simulink model "VCOs"  (R2019b)
settings: Solver=FixedStepAuto  StartTime=0.0  StopTime=simt  FixedStep=sampt  RelTol=1e-3
model workspace (MAT data in the model file):
  VCOctrl = 1
  Vc = 2.421875
  VcoParamResultTable = [nan nan]
  frequencyVector = [nan nan nan nan nan nan nan nan nan nan]
  kvcoVector = [nan nan nan nan nan nan nan nan nan]
  myParam = Simulink.Parameter
  myParam.Value = 2
  myParam.DataType = 'auto'
  myParam.Min = 0
  myParam.Max = 5
  myParam.Dimensions = [1 1]
  myParam2 = 2
  quiescentFreq = nan
  vctrlVector = [1 1.44 1.89 2.33 2.78 3.22 3.67 4.11 4.56 5]
values from neighbouring files (symbols this model uses):
  simt = 1/100000    (= 1e-05)    [FreqSpectrum.m]    (also in VCO.m)
libraries: impairlib x1, simulink x1, msbPllFoundation x1
settings Model: OrderedModelArguments=off  Creator=lfbarrag  LastModifiedBy=Luis Barragan
settings DataIOCC: SaveFormat=Array  ReturnWorkspaceOutputs=off

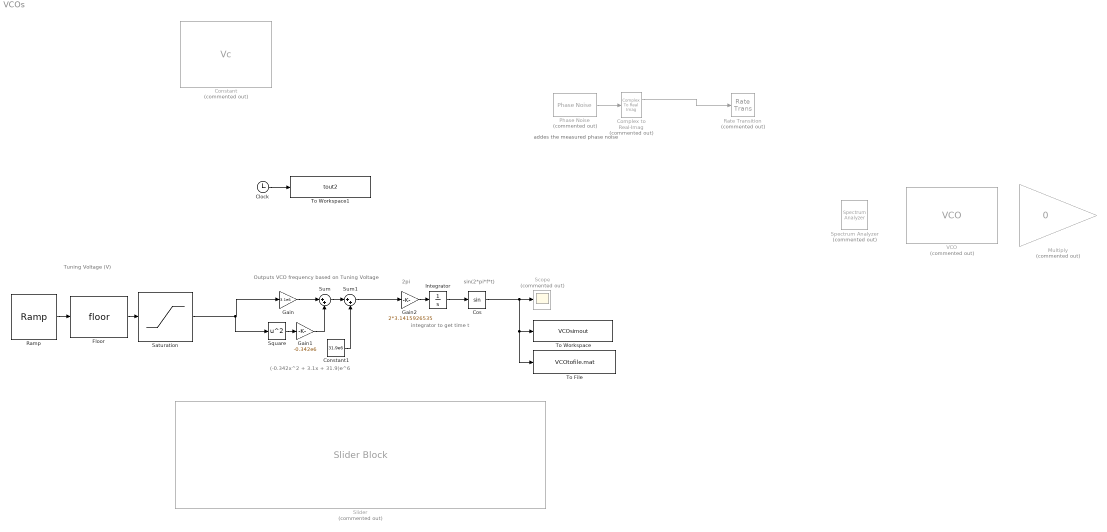
== system VCOs ==
  note: (-0.342x^2 + 3.1x + 31.9)e^6
  note: addes the measured phase noise
  note: Outputs VCO frequency based on Tuning Voltage
  note: integrator to get time t
  note: Tuning Voltage
      | (V)
  note: 2pi
  note: sin(2*pi*f*t)
  Clock : Clock
  Complex to Real-Imag : ComplexToRealImag  Commented=on
  Constant : Constant  Commented=on  Value=Vc  OutMin=[0]  OutMax=[5]
  Constant1 : Constant  Value=31.9e6
  Cos : Trigonometry  OutputSignalType=complex
  Floor : Rounding
  Gain : Gain  Gain=3.1e6
  Gain1 : Gain  Gain=-0.342e6
  Gain2 : Gain  Gain=2*3.1415926535
  Integrator : Integrator
  Multiply : Gain  Commented=on  Gain=0
  Phase Noise : impairlib/Phase Noise  Commented=on  Level=[ -36, -73, -83, -90, -112 ]  FrequencyOffset=[ 100, 400, 1000, 5000, 250000]  SampleRate=550000  RandomStream=mt19937ar with seed  Seed=1e6  SimulateUsing=Interpreted execution
      settings: SourceProductName=SerDes Toolbox  SourceProductBaseCode=SX
  Ramp : simulink/Sources/Ramp  slope=5/simt  start=0  InitialOutput=0
  Rate Transition : RateTransition  Commented=on  OutPortSampleTime=1e-9
  Saturation : Saturate  UpperLimit=5  LowerLimit=0
  Scope : Scope  Commented=on
  Slider : SliderBlock  Commented=on  ScaleMax=5  TickInterval=.1
  Spectrum Analyzer : SpectrumAnalyzer  Commented=on
  Square : Math  Operator=square  SignedPower=off  SaturateOnIntegerOverflow=on
  Sum : Sum  Inputs=|++
  Sum1 : Sum  Inputs=|++
  To File : ToFile  Filename=VCOtofile.mat  MatrixName=VCOtofile  SaveFormat=Timeseries
  To Workspace : ToWorkspace  VariableName=VCOsimout  SampleTime=-1
      settings: Save2DSignal=2-D array (concatenate along first dimension)
  To Workspace1 : ToWorkspace  VariableName=tout2  SampleTime=-1
      settings: Save2DSignal=2-D array (concatenate along first dimension)
  VCO : msbPllFoundation/VCO  Commented=on  SpecifyUsing=Voltage sensitivity  Kvco=1.4e0  Fo=32.1e6  ControlVoltage=[1 5]  OutputFrequency=[25e6 35e6]  Amplitude=1  ExtraBuffer=off  NBuffer=10  AddPhaseNoise=off  Foffset=[100 200 300 400 1000 2000 5000 100000 250000]  PhaseNoise=[-35.8 -65 -70 -72.9 -83.4 -89 -90.1 -96.5 -111.6]  MaxKvco=1.4
      settings: SourceProductName=Mixed-Signal Blockset  SourceProductBaseCode=AM
  wires:
  Complex to Real-Imag/1 -> Rate Transition/1
  Phase Noise/1 -> Complex to Real-Imag/1
  Sum/1 -> Sum1/1
  Sum1/1 -> Gain2/1
  Square/1 -> Gain1/1
  Gain1/1 -> Sum/2
  Gain2/1 -> Integrator/1
  Constant1/1 -> Sum1/2
  Integrator/1 -> Cos/1
  Gain/1 -> Sum/1
  Cos/1 -> To File/1, To Workspace/1, Scope/1
  Saturation/1 -> Square/1, Gain/1
  Ramp/1 -> Floor/1
  Floor/1 -> Saturation/1
  Clock/1 -> To Workspace1/1
